simulink model "Model_3_Flux_weakening_control"  (R2017b)
settings: Solver=VariableStepAuto  StartTime=0.0  StopTime=5  MaxStep=1e-4  RelTol=1e-3  EnableMultiTasking=on
values from neighbouring files (symbols this model uses):
  Gain_I = 1    [Model_1_init.m]    (also in Model_2_init.m = 26.84; Model_3_init.m = 26.84)
  Gain_P = 1    [Model_1_init.m]    (also in Model_2_init.m = 7.74; Model_3_init.m = 7.74)
  Lambda_m = 0.2205    [Model_1_init.m]    (also in Model_2_init.m; Model_3_init.m)
  Ld = 1.7e-3    (= 0.0017)    [Model_1_init.m]    (also in Model_2_init.m; Model_3_init.m)
  Lq = 3.2e-3    (= 0.0032)    [Model_1_init.m]    (also in Model_2_init.m; Model_3_init.m)
  Param_BaseSpeed = 876    [Model_3_init.m]
  Param_Id_of_We_Torque = [0,-2.30177543036769,-8.59356944788153,-16.4990590457644,-24.2019970239658,-31.7336385477141,-39.1248735240059,-46.3895339353480,-53.5438693452557,-60.5877368527563,-67.5279121716960,-74.3632914076158,-81.0848264560473,-87.6900840096281,-94.1727155294297,-100.524695788491,-106.737943081073,-112.804868607954,-118.718887132852,-124.474863382221,-130.069470306117,-135.501440241541,-140.771697570859,- ...(+15575 chars)    [Model_3_init.m]
  Param_Iq_of_We_Torque = [0,17.4374754938312,33.6052724806698,47.9620946336906,61.0927552487034,73.1479215327095,84.3049660756008,94.6583419249824,104.337724889008,113.390978591554,121.917651973936,129.979877833255,137.614541014493,144.885610404097,151.839336396392,158.514190867132,164.945264651086,171.164425441937,177.200422756775,183.078971644055,188.822841517577,194.451970162672,199.983615838069,205.431863624177,210.80 ...(+14449 chars)    [Model_3_init.m]
  ParamControlTableTrqIndex = [0,23.5444010560252,47.0888021120504,70.6332031680755,94.1776042241007,117.722005280126,141.266406336151,164.810807392176,188.355208448201,211.899609504227,235.444010560252,258.988411616277,282.532812672302,306.077213728327,329.621614784353,353.166015840378,376.710416896403,400.254817952428,423.799219008453,447.343620064478,470.888021120504,494.432422176529,517.976823232554,541.521224288579,565.06 ...(+113 chars)    [Model_3_init.m]
  ParamControlTableWeIndex = [875.837524774747,1058.84332746136,1241.84913014798,1424.85493283460,1607.86073552121,1790.86653820783,1973.87234089444,2156.87814358106,2339.88394626768,2522.88974895429,2705.89555164091,2888.90135432753,3071.90715701414,3254.91295970076,3437.91876238737,3620.92456507399,3803.93036776061,3986.93617044722,4169.94197313384,4352.94777582045,4535.95357850707,4718.95938119369,4901.96518388030,5084.970 ...(+82 chars)    [Model_3_init.m]
  Polepairs = 4    [Model_1_init.m]    (also in Model_2_init.m; Model_3_init.m)
  Rs = 0.02    [Model_1_init.m]    (also in Model_2_init.m; Model_3_init.m)
undefined symbols (not defined in the file or in its folder): sigbuilder_block
libraries: powerlib x18, simulink x5, powerlib_meascontrol x1
settings Model: SimulationMode=accelerator  Creator=dakaihu  LastModifiedBy=proso
settings DataIOCC: LimitDataPoints=on
settings OptimizationCC: LifeSpan=inf
settings DebuggingCC: AllowSymbolicDim=off  SFUnexpectedBacktrackingDiag=warning  SFNoUnconditionalDefaultTransitionDiag=warning  SFExecutionAtInitializationDiag=none
settings ModelReferenceCC: PropagateSignalLabelsOutOfModel=off
settings CodeAppCC: StateflowObjectComments=on
settings GRTTargetCC: TargetLangStandard=C89/C90 (ANSI)
settings ConfigComp: CovMetricSettings=dw  CovSaveCumulativeToWorkspaceVar=on  CovSaveSingleToWorkspaceVar=on  CovExternalEMLEnable=off
settings SimscapeCC: SimscapeNormalizeSystem=off

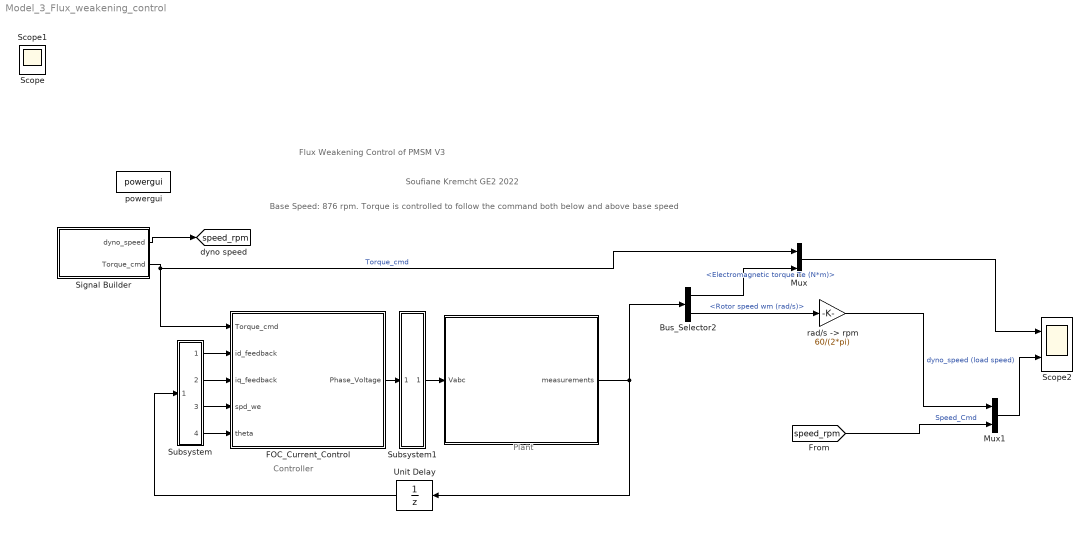
== system Model_3_Flux_weakening_control ==
  note: Soufiane Kremcht GE2 2022
  note: Base Speed: 876 rpm. Torque is controlled to follow the command both below and above base speed
  note: Controller
  note: Plant
  note: Flux Weakening Control of PMSM V3
  " " : Subsystem
  Bus_Selector2 : BusSelector  OutputSignals=Electromagnetic torque Te (N*m),Rotor speed wm (rad/s)
  FOC_Current_Control : Subsystem
  Mux : Mux  Inputs=2
  Mux1 : Mux  Inputs=2
  Scope2 : Scope  NumInputPorts=2
  Signal Builder : Subsystem  Tag=STV Subsys  LoadFcn=sigbuilder_block('load',[326.4 117 550.8 361.8 ]);  StartFcn=sigbuilder_block('start');  StopFcn=sigbuilder_block('stop');  ClipboardFcn=sigbuilder_block('clipboard');  mask(Sigbuilder block){tuvar=[0:10]}
      mask help: Simulink:masks:SigbuilderBlock_MD
      mask init:
      | if ~strcmp(get_param(bdroot(gcbh),'SimulationStatus'),'stopped') tuvar = sigbuilder_block('maskInit'); end
      settings: CopyFcn=sigbuilder_block('copy');  DeleteFcn=sigbuilder_block('delete');  ModelCloseFcn=sigbuilder_block('modelClose');  PreSaveFcn=sigbuilder_block('preSave');  PauseFcn=sigbuilder_block('pause');  ContinueFcn=sigbuilder_block('continue');  NameChangeFcn=sigbuilder_block('namechange');  OpenFcn=sigbuilder_block('open',[326.4 117 550.8 361.8 ]);  CloseFcn=sigbuilder_block('close');
      mask Display: plot(0, 0, 100, 100,[2, 2, 32, 32, 2], [68, 8, 8, 68, 68],[32, 2], [38, 38], [32, 19, 2],[53, 60, 44], [32, 17, 17, 2],[16, 16, 31, 31]);txt = getActiveGroup(gcbh);text(2, 100, txt,'verticalAlignment', 'top');
  Subsystem : Subsystem
      mask Display: fprintf('C/D')
  Subsystem1 : Subsystem
      mask Display: fprintf('D/C')
  Unit Delay : UnitDelay  SampleTime=1e-4
  powergui : powerlib/powergui  SimulationMode=Continuous  SampleTime=1e-5  frequency=60  Iterations=50  frequencyindice=0  Pbase=100e6  ErrMax=1e-4  UnitsV=kV  UnitsW=MW  buscounter=0  FunctionMessages=off  echomessages=off  EnableUseOfTLC=off  CurrentSourceSwitches=off  DisableSnubberDevices=off  DisableRonSwitches=off  DisableVfSwitches=off  DisplayEquations=off  SolverType=Tustin/Backward Euler (TBE)  Interpol=off  ExternalGateDelay=off  methode=off  Ts=100  x0status=blocks  SPID=on  SwTol=0  HookPort=off  RestoreLinks=warning  ResistiveCurrentMeasurement=off  Frange=[0:2:500]  Ylog=off  Xlog=on  ShowGrid=off  save=off  variable=ZData  structure=0  ZoomFFT=on  StartTime=0.0  cycles=1  DisplayStyle=1  fundamental=60  FreqAxis=off  MaxFrequency=1000  frequencyindicesteady=1  RmsSteady=1  display=off
  "rad/s -> rpm" : Gain  Gain=60/(2*pi)
  Scope : Scope
  Scope1 : Scope
  tag scope: speed_rpm=global
  wires:
  FOC_Current_Control/1(Phase_Voltage) -> Subsystem1/1(In1)
  " "/1(measurements) -> Unit Delay/1, Bus_Selector2/1
  Subsystem1/1(Out1) -> " "/1(Vabc)
  Unit Delay/1 -> Subsystem/1(PMSM_Measurements)
  Mux/1 -> Scope2/1
  Bus_Selector2/1 -> Mux/2  "<Electromagnetic torque Te (N*m)>"
  Subsystem/1(Out2) -> FOC_Current_Control/2(id_feedback)
  Subsystem/2(Out3) -> FOC_Current_Control/3(iq_feedback)
  Subsystem/3(Out1) -> FOC_Current_Control/4(spd_we)
  Subsystem/4(Out4) -> FOC_Current_Control/5(theta)
  Signal Builder/2(Torque_cmd) -> FOC_Current_Control/1(Torque_cmd), Mux/1  "Torque_cmd"
  Signal Builder/1(dyno_speed) -> [speed_rpm]
  Bus_Selector2/2 -> "rad/s -> rpm"/1  "<Rotor speed wm (rad/s)>"
  [speed_rpm] -> Mux1/2  "Speed_Cmd"
  "rad/s -> rpm"/1 -> Mux1/1  "dyno_speed (load speed)"
  Mux1/1 -> Scope2/2

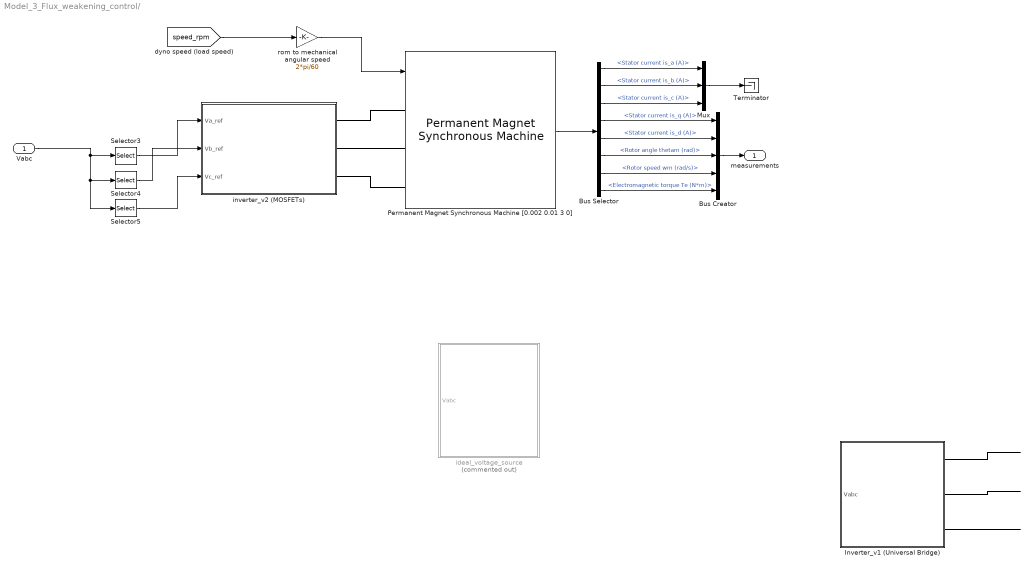
== system Model_3_Flux_weakening_control/  ==
  Vabc : Inport
  " Inverter_v1 (Universal Bridge)" : Subsystem
  Bus Creator : BusCreator  Inputs=5
  Bus Selector : BusSelector  OutputSignals=Stator current is_a (A),Stator current is_b (A),Stator current is_c (A),Stator current is_q (A),Stator current is_d (A),Rotor angle thetam (rad),Rotor speed wm (rad/s),Electromagnetic torque Te (N*m)
  Mux : Mux  Inputs=3
  Permanent Magnet Synchronous Machine [0.002 0.01 3 0] : powerlib/Machines/Permanent Magnet Synchronous Machine  NbPhases=3  FluxDistribution=Sinusoidal  RotorType=Salient-pole  MechanicalLoad=Speed w  PresetModel=No  ShowDetailedParameters=on  MeasurementBus=off  Resistance=Rs  Inductance=8.5e-3  dqInductances=[Ld,Lq]  La=0.000395  MachineConstant=Flux linkage established by magnets (V.s)  Flux=Lambda_m  VoltageCst=159.9771  TorqueCst=1.323  Flat=120  Mechanical=[0.0027 0.001 4 0]  PolePairs=Polepairs  InitialConditions=[0,0, 0,0]  InitialConditions5ph=[0 0 0 0 0 0]  TsPowergui=0  TsBlock=-1  RefAngle=Aligned with phase A axis (original Park)
  Selector3 : Selector  InputPortWidth=3  IndexOptions=Index vector (dialog)  Indices=[1]  OutputSizes=1
  Selector4 : Selector  InputPortWidth=3  IndexOptions=Index vector (dialog)  Indices=2  OutputSizes=1
  Selector5 : Selector  InputPortWidth=3  IndexOptions=Index vector (dialog)  Indices=3  OutputSizes=1
  Terminator : Terminator
  ideal_voltage_source : Subsystem  Commented=on  VariantControl=variantPwm == enumPwm.behavior
  inverter_v2 (MOSFETs) : Subsystem
  rom to mechanical angular speed : Gain  Gain=2*pi/60
  measurements : Outport
  wires:
  rom to mechanical angular speed/1 -> Permanent Magnet Synchronous Machine [0.002 0.01 3 0]/1
  Bus Selector/4 -> Bus Creator/1  "<Stator current is_q (A)>"
  Bus Selector/5 -> Bus Creator/2  "<Stator current is_d (A)>"
  Bus Selector/6 -> Bus Creator/3  "<Rotor angle thetam (rad)>"
  Bus Creator/1 -> measurements/1
  Bus Selector/1 -> Mux/1  "<Stator current is_a (A)>"
  Bus Selector/2 -> Mux/2  "<Stator current is_b (A)>"
  Bus Selector/3 -> Mux/3  "<Stator current is_c (A)>"
  Mux/1 -> Terminator/1
  Permanent Magnet Synchronous Machine [0.002 0.01 3 0]/1 -> Bus Selector/1
  Bus Selector/7 -> Bus Creator/4  "<Rotor speed wm (rad/s)>"
  [speed_rpm] -> rom to mechanical angular speed/1
  Bus Selector/8 -> Bus Creator/5  "<Electromagnetic torque Te (N*m)>"
  Vabc/1 -> Selector5/1, Selector4/1, Selector3/1
  Selector3/1 -> inverter_v2 (MOSFETs)/1(Va_ref)
  Selector4/1 -> inverter_v2 (MOSFETs)/2(Vb_ref)
  Selector5/1 -> inverter_v2 (MOSFETs)/3(Vc_ref)
  connections:
  " Inverter_v1 (Universal Bridge)"/RConn3 -- ?
  " Inverter_v1 (Universal Bridge)"/RConn2 -- ?
  " Inverter_v1 (Universal Bridge)"/RConn1 -- ?
  inverter_v2 (MOSFETs)/RConn1 -- Permanent Magnet Synchronous Machine [0.002 0.01 3 0]/LConn1
  inverter_v2 (MOSFETs)/RConn2 -- Permanent Magnet Synchronous Machine [0.002 0.01 3 0]/LConn2
  inverter_v2 (MOSFETs)/RConn3 -- Permanent Magnet Synchronous Machine [0.002 0.01 3 0]/LConn3

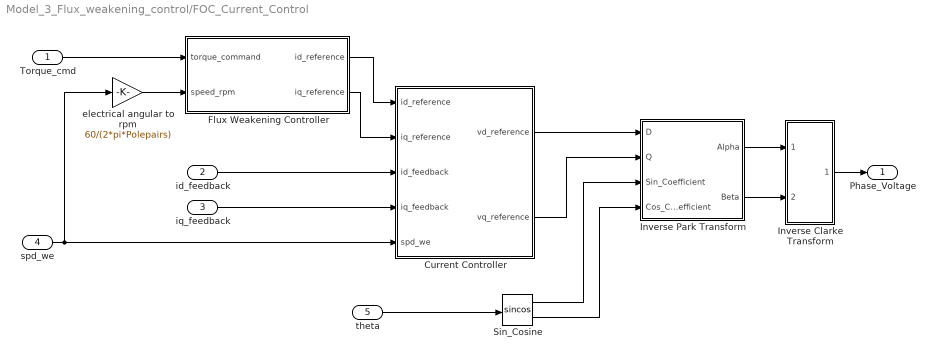
== system Model_3_Flux_weakening_control/FOC_Current_Control ==
  Torque_cmd : Inport
  id_feedback : Inport  Port=2
  iq_feedback : Inport  Port=3
  spd_we : Inport  Port=4
  theta : Inport  Port=5
  Current Controller : Subsystem
  Flux Weakening Controller : Subsystem
  Inverse Clarke Transform : Subsystem
  Inverse Park Transform : Subsystem
  Sin_Cosine : Trigonometry  Operator=sincos
  electrical angular to rpm : Gain  Gain=60/(2*pi*Polepairs)
  Phase_Voltage : Outport  SampleTime=1e-4
  wires:
  Inverse Clarke Transform/1(ABC) -> Phase_Voltage/1
  Sin_Cosine/2 -> Inverse Park Transform/4(Cos_Coefficient)
  Sin_Cosine/1 -> Inverse Park Transform/3(Sin_Coefficient)
  theta/1 -> Sin_Cosine/1
  Current Controller/2(vq_reference) -> Inverse Park Transform/2(Q)
  Current Controller/1(vd_reference) -> Inverse Park Transform/1(D)
  Inverse Park Transform/1(Alpha) -> Inverse Clarke Transform/1(Alpha)
  Inverse Park Transform/2(Beta) -> Inverse Clarke Transform/2(Beta)
  Flux Weakening Controller/1(id_reference) -> Current Controller/1(id_reference)
  Flux Weakening Controller/2(iq_reference) -> Current Controller/2(iq_reference)
  Torque_cmd/1 -> Flux Weakening Controller/1(torque_command)
  spd_we/1 -> Current Controller/5(spd_we), electrical angular to rpm/1
  electrical angular to rpm/1 -> Flux Weakening Controller/2(speed_rpm)
  id_feedback/1 -> Current Controller/3(id_feedback)
  iq_feedback/1 -> Current Controller/4(iq_feedback)

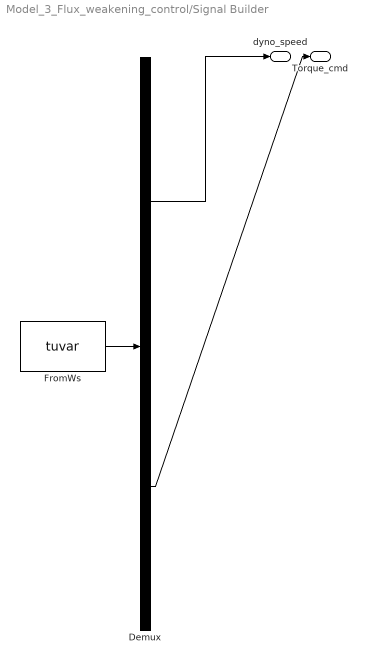
== system Model_3_Flux_weakening_control/Signal Builder ==
  Demux : Demux  Tag=STV Demux  Outputs=2
  FromWs : FromWorkspace  Tag=STV FromWs  VariableName=tuvar  SampleTime=0
      SigBuilderData=|
      | common.afterFinalStr = 'Extrapolate'
      | common.sampleTime = 0
      | dataSet.timeRange = [0 3]
      | dataSet.name = 'Group 1'
      | sbobj.Groups.Name = 'Group 1'
      | sbobj.Groups.Signals(1).Name = 'dyno_speed'
      | sbobj.Groups.Signals(1).XData = [0 1 2 3]
      | sbobj.Groups.Signals(1).YData = [0 1500 1500 -20]
      | sbobj.Groups.Signals(2).Name = 'Torque_cmd'
      | sbobj.Groups.Signals(2).XData = [0 0.995 0.995 3]
      | sbobj.Groups.Signals(2).YData = [100 98 218 218]
      | sbobj.Groups.TimeRange = [0 3]
  dyno_speed : Outport  Tag=STV Outport
  Torque_cmd : Outport  Tag=STV Outport  Port=2
  wires:
  Demux/1 -> dyno_speed/1
  FromWs/1 -> Demux/1
  Demux/2 -> Torque_cmd/1

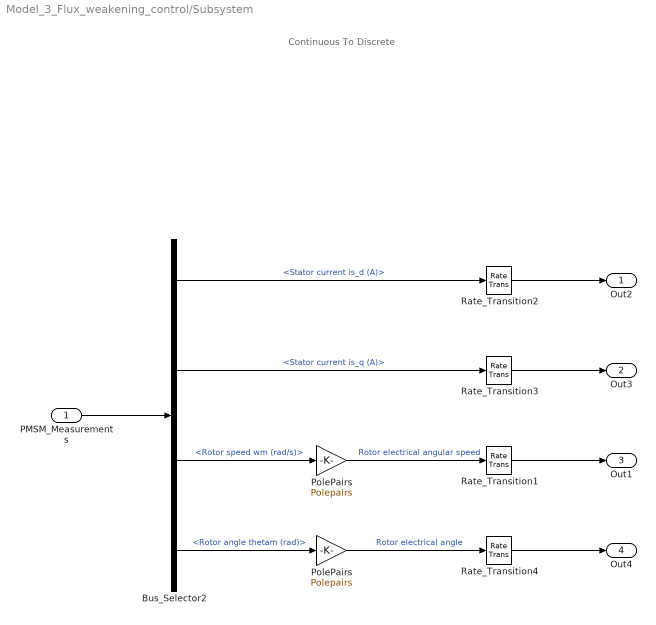
== system Model_3_Flux_weakening_control/Subsystem ==
  note: Continuous To Discrete
  PMSM_Measurements : Inport
  Bus_Selector2 : BusSelector  OutputSignals=Stator current is_d (A),Stator current is_q (A),Rotor speed wm (rad/s),Rotor angle thetam (rad)
  PolePairs : Gain  Gain=Polepairs
  "PolePairs " : Gain  Gain=Polepairs
  Rate_Transition{1..4} (4 alike) : RateTransition  Integrity=off  Deterministic=off
  Out2 : Outport
  Out3 : Outport  Port=2
  Out1 : Outport  Port=3
  Out4 : Outport  Port=4
  wires:
  Rate_Transition4/1 -> Out4/1
  Bus_Selector2/4 -> PolePairs/1  "<Rotor angle thetam (rad)>"
  PMSM_Measurements/1 -> Bus_Selector2/1
  PolePairs/1 -> Rate_Transition4/1  "Rotor electrical angle"
  Rate_Transition2/1 -> Out2/1
  Rate_Transition3/1 -> Out3/1
  Rate_Transition1/1 -> Out1/1
  Bus_Selector2/3 -> "PolePairs "/1  "<Rotor speed wm (rad/s)>"
  "PolePairs "/1 -> Rate_Transition1/1  "Rotor electrical angular speed"
  Bus_Selector2/1 -> Rate_Transition2/1  "<Stator current is_d (A)>"
  Bus_Selector2/2 -> Rate_Transition3/1  "<Stator current is_q (A)>"

== system Model_3_Flux_weakening_control/Subsystem1 ==
  In1 : Inport
  Rate_Transition1 : RateTransition  Integrity=off
  Out1 : Outport
  wires:
  In1/1 -> Rate_Transition1/1
  Rate_Transition1/1 -> Out1/1

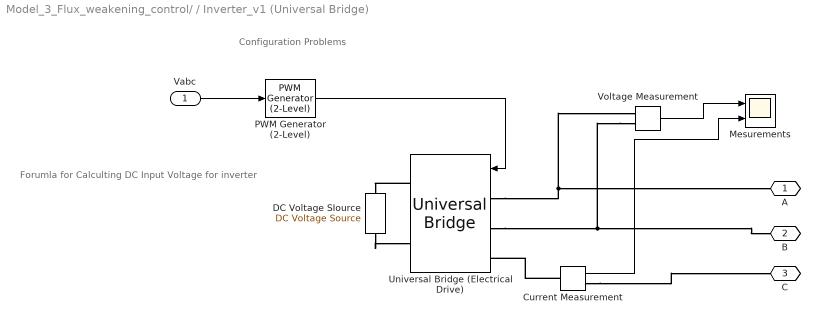
== system Model_3_Flux_weakening_control/ / Inverter_v1 (Universal Bridge) ==
  note: Forumla for Calculting DC Input Voltage for inverter
  note: Configuration Problems
  Vabc : Inport
  Current Measurement : powerlib/Measurements/Current Measurement  PhasorSimulation=off  OutputType=Complex  PSBequivalent=0
  DC Voltage SIource : powerlib/Electrical Sources/DC Voltage Source  Amplitude=320  Measurements=None
  Mesurements : Scope  NumInputPorts=2
  PWM Generator (2-Level) : powerlib_meascontrol/Pulse & Signal Generators/PWM Generator (2-Level)  ModulatorType=Three-phase bridge (6 pulses)  ModulatorMode=Unsynchronized  Fc=27*60  Pc=90  nF=27  MinMax="[ -1  1 ]"  SamplingTechnique=Natural  ModulatingSignals=off  m=0.8  Freq=60  Phase=0  Ts=0  ShowCarrierOutport=off
      settings: SourceProductName=Simscape Power Systems
  Universal Bridge (Electrical Drive) : powerlib/Power Electronics/Universal Bridge  Arms=3  SnubberResistance=1e5  SnubberCapacitance=inf  Device=IGBT / Diodes  Ron=1e-2  Lon=0  ForwardVoltages="[  0  0  ]"  ForwardVoltage=0  GTOparameters=[ 10e-6 , 20e-6 ]  IGBTparameters=[ 1e-6 , 2e-6 ]  Measurements=None  Measurements_2=None  converterType=Rectifier
  Voltage Measurement : powerlib/Measurements/Voltage Measurement  PhasorSimulation=off  OutputType=Complex  PSBequivalent=0
  A : PMIOPort  Port=1  Side=Right
  B : PMIOPort  Port=2  Side=Right
  C : PMIOPort  Port=3  Side=Right
  wires:
  PWM Generator (2-Level)/1 -> Universal Bridge (Electrical Drive)/1
  Vabc/1 -> PWM Generator (2-Level)/1
  Voltage Measurement/1 -> Mesurements/1
  Current Measurement/1 -> Mesurements/2
  connections:
  Universal Bridge (Electrical Drive)/RConn1 -- DC Voltage SIource/RConn1
  DC Voltage SIource/LConn1 -- Universal Bridge (Electrical Drive)/RConn2
  Current Measurement/LConn1 -- Universal Bridge (Electrical Drive)/LConn3
  Universal Bridge (Electrical Drive)/LConn1 -- Voltage Measurement/LConn1 -- A/RConn1
  Voltage Measurement/LConn2 -- Universal Bridge (Electrical Drive)/LConn2 -- B/RConn1
  Current Measurement/RConn1 -- C/RConn1

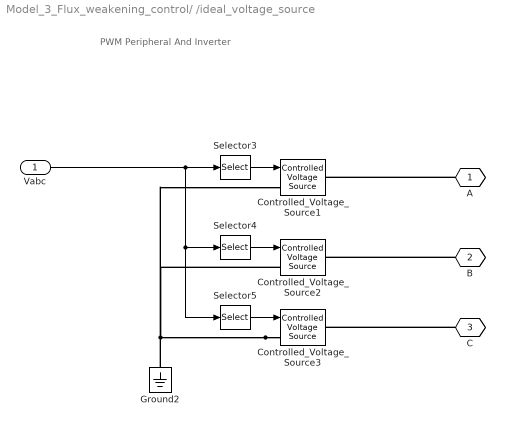
== system Model_3_Flux_weakening_control/ /ideal_voltage_source ==
  note: PWM Peripheral And Inverter
  Vabc : Inport
  Controlled_Voltage_Source1 : powerlib/Electrical Sources/Controlled Voltage Source  Initialize=off  Source_Type=DC  Amplitude=12  Phase=0  Frequency=0  Measurements=None
  Controlled_Voltage_Source2 : powerlib/Electrical Sources/Controlled Voltage Source  Initialize=off  Source_Type=DC  Amplitude=12  Phase=0  Frequency=0  Measurements=None
  Controlled_Voltage_Source3 : powerlib/Electrical Sources/Controlled Voltage Source  Initialize=off  Source_Type=DC  Amplitude=12  Phase=0  Frequency=0  Measurements=None
  Ground2 : powerlib/Elements/Ground  LConnTagsString=a
  Selector3 : Selector  InputPortWidth=3  IndexOptions=Index vector (dialog)  Indices=[1]  OutputSizes=1
  Selector4 : Selector  InputPortWidth=3  IndexOptions=Index vector (dialog)  Indices=2  OutputSizes=1
  Selector5 : Selector  InputPortWidth=3  IndexOptions=Index vector (dialog)  Indices=3  OutputSizes=1
  A : PMIOPort  Tag=PMCPort  Port=1  Side=Right
  B : PMIOPort  Tag=PMCPort  Port=2  Side=Right
  C : PMIOPort  Tag=PMCPort  Port=3  Side=Right
  wires:
  Vabc/1 -> Selector4/1, Selector5/1, Selector3/1
  Selector5/1 -> Controlled_Voltage_Source3/1
  Selector4/1 -> Controlled_Voltage_Source2/1
  Selector3/1 -> Controlled_Voltage_Source1/1
  connections:
  C/RConn1 -- Controlled_Voltage_Source3/RConn1
  B/RConn1 -- Controlled_Voltage_Source2/RConn1
  A/RConn1 -- Controlled_Voltage_Source1/RConn1
  Controlled_Voltage_Source3/LConn1 -- Controlled_Voltage_Source1/LConn1 -- Controlled_Voltage_Source2/LConn1 -- Ground2/LConn1

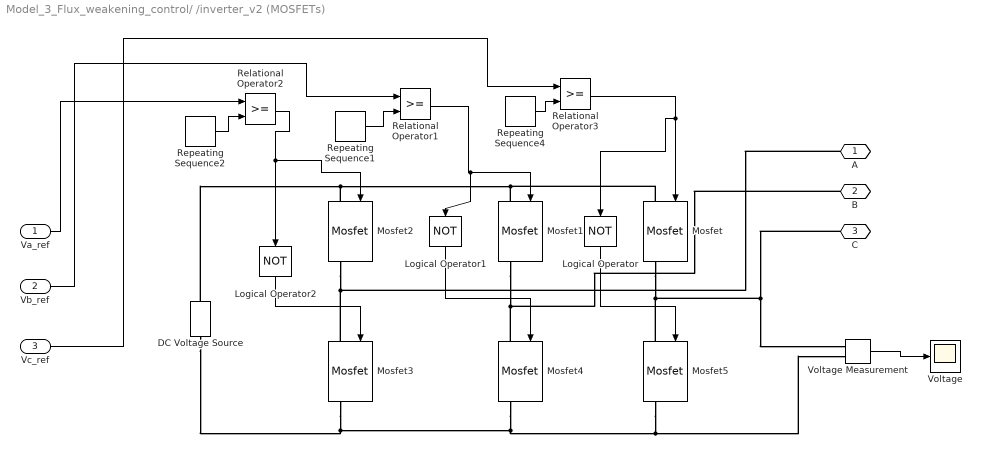
== system Model_3_Flux_weakening_control/ /inverter_v2 (MOSFETs) ==
  Va_ref : Inport
  Vb_ref : Inport  Port=2
  Vc_ref : Inport  Port=3
  DC Voltage Source : powerlib/Electrical Sources/DC Voltage Source  Amplitude=320  Measurements=None
  Logical Operator : Logic  Operator=NOT  AllPortsSameDT=off  OutDataTypeStr=boolean
  Logical Operator1 : Logic  Operator=NOT  AllPortsSameDT=off  OutDataTypeStr=boolean
  Logical Operator2 : Logic  Operator=NOT  AllPortsSameDT=off  OutDataTypeStr=boolean
  Mosfet{,1..5} (6 alike) : powerlib/Power Electronics/Mosfet  Ron=0.1  Lon=0  Rd=0.01  Vfd=0  IC=0  Rs=1e5  Cs=inf  Measurements=on
  Relational Operator1 : RelationalOperator  OutDataTypeStr=boolean  RndMeth=Simplest
  Relational Operator2 : RelationalOperator  OutDataTypeStr=boolean  RndMeth=Simplest
  Relational Operator3 : RelationalOperator  OutDataTypeStr=boolean  RndMeth=Simplest
  Repeating Sequence1 : simulink/Sources/Repeating Sequence  rep_seq_t="[0 (1/5000)/4  (1/5000)/2 (3/5000)/4 1/5000]"  rep_seq_y=[0 1 0 -1 0]
  Repeating Sequence2 : simulink/Sources/Repeating Sequence  rep_seq_t="[0 (1/5000)/4  (1/5000)/2 (3/5000)/4 1/5000]"  rep_seq_y=[0 1 0 -1 0]
  Repeating Sequence4 : simulink/Sources/Repeating Sequence  rep_seq_t="[0 (1/5000)/4  (1/5000)/2 (3/5000)/4 1/5000]"  rep_seq_y=[0 1 0 -1 0]
  Voltage : Scope
  Voltage Measurement : powerlib/Measurements/Voltage Measurement  PhasorSimulation=off  OutputType=Complex  PSBequivalent=0
  A : PMIOPort  Port=1  Side=Right
  B : PMIOPort  Port=2  Side=Right
  C : PMIOPort  Port=3  Side=Right
  wires:
  Relational Operator1/1 -> Mosfet1/1, Logical Operator1/1
  Vc_ref/1 -> Relational Operator3/1
  Logical Operator2/1 -> Mosfet3/1
  Va_ref/1 -> Relational Operator2/1
  Repeating Sequence4/1 -> Relational Operator3/2
  Repeating Sequence2/1 -> Relational Operator2/2
  Repeating Sequence1/1 -> Relational Operator1/2
  Relational Operator3/1 -> Mosfet/1, Logical Operator/1
  Relational Operator2/1 -> Mosfet2/1, Logical Operator2/1
  Vb_ref/1 -> Relational Operator1/1
  Logical Operator/1 -> Mosfet5/1
  Logical Operator1/1 -> Mosfet4/1
  Voltage Measurement/1 -> Voltage/1
  connections:
  Mosfet2/LConn1 -- Mosfet1/LConn1 -- Mosfet/LConn1 -- DC Voltage Source/RConn1
  Mosfet5/LConn1 -- Mosfet/RConn1 -- C/RConn1 -- Voltage Measurement/LConn1
  Mosfet3/LConn1 -- Mosfet2/RConn1 -- A/RConn1
  Mosfet5/RConn1 -- DC Voltage Source/LConn1 -- Mosfet3/RConn1 -- Mosfet4/RConn1 -- Voltage Measurement/LConn2
  Mosfet4/LConn1 -- Mosfet1/RConn1 -- B/RConn1

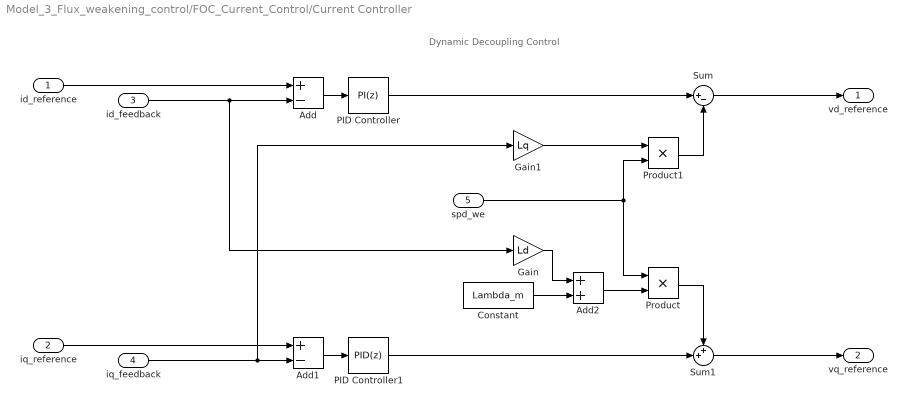
== system Model_3_Flux_weakening_control/FOC_Current_Control/Current Controller ==
  note: Dynamic Decoupling Control
  id_reference : Inport  SampleTime=1e-4
  iq_reference : Inport  Port=2  SampleTime=1e-4
  id_feedback : Inport  Port=3  SampleTime=1e-4
  iq_feedback : Inport  Port=4  SampleTime=1e-4
  spd_we : Inport  Port=5  SampleTime=1e-4
  Add : Sum  Inputs=+-
  Add1 : Sum  Inputs=+-
  Add2 : Sum
  Constant : Constant  Value=Lambda_m  SampleTime=1e-4
  Gain : Gain  Gain=Ld
  Gain1 : Gain  Gain=Lq
  PID Controller : simulink/Continuous/PID Controller  Controller=PI  TimeDomain=Discrete-time  SampleTime=-1  IntegratorMethod=Forward Euler  FilterMethod=Forward Euler  Form=Parallel  UseFilter=on  ControllerParametersSource=internal  P=Gain_P  I=Gain_I  D=0  N=100  InitialConditionSource=internal  InitialConditionForIntegrator=0  InitialConditionForFilter=0  ExternalReset=none  LimitOutput=off  UpperSaturationLimit=inf  LowerSaturationLimit=-inf  LinearizeAsGain=on  AntiWindupMode=none  Kb=1  TrackingMode=off  Kt=1  PParamMin=[]  PParamMax=[]  IParamMin=[]  IParamMax=[]  DParamMin=[]  DParamMax=[]  NParamMin=[]  NParamMax=[]  KbParamMin=[]  KbParamMax=[]  KtParamMin=[]  KtParamMax=[]  POutMin=[]  POutMax=[]  IOutMin=[]  IOutMax=[]  DOutMin=[]  DOutMax=[]  NOutMin=[]  NOutMax=[]  KbOutMin=[]  KbOutMax=[]  KtOutMin=[]  KtOutMax=[]  IntegratorOutMin=[]  IntegratorOutMax=[]  FilterOutMin=[]  FilterOutMax=[]  SumOutMin=[]  SumOutMax=[]  SumI1OutMin=[]  SumI1OutMax=[]  SumI2OutMin=[]  SumI2OutMax=[]  SumI3OutMin=[]  SumI3OutMax=[]  SumDOutMin=[]  SumDOutMax=[]  SaturationOutMin=[]  SaturationOutMax=[]  IntegratorContinuousStateAttributes=''  IntegratorStateMustResolveToSignalObject=off  IntegratorRTWStateStorageClass=Auto  FilterContinuousStateAttributes=''  FilterStateMustResolveToSignalObject=off  FilterRTWStateStorageClass=Auto  DifferentiatorICPrevScaledInput=0  DifferentiatorOutMin=[]  DifferentiatorOutMax=[]  InitialConditionSetting=State (most efficient)  FilterDiffOutCoefMin=[]  FilterDiffOutCoefMax=[]  SumDenOutMin=[]  SumDenOutMax=[]  SumNumOutMin=[]  SumNumOutMax=[]  ReciprocalOutMin=[]  ReciprocalOutMax=[]  DivideOutMin=[]  DivideOutMax=[]  TunerSelectOption=Transfer Function Based (PID Tuner App)
  PID Controller1 : simulink/Continuous/PID Controller  Controller=PID  TimeDomain=Discrete-time  SampleTime=-1  IntegratorMethod=Forward Euler  FilterMethod=Forward Euler  Form=Parallel  UseFilter=on  ControllerParametersSource=internal  P=Gain_P  I=Gain_I  D=0  N=100  InitialConditionSource=internal  InitialConditionForIntegrator=0  InitialConditionForFilter=0  ExternalReset=none  LimitOutput=off  UpperSaturationLimit=inf  LowerSaturationLimit=-inf  LinearizeAsGain=on  AntiWindupMode=none  Kb=1  TrackingMode=off  Kt=1  PParamMin=[]  PParamMax=[]  IParamMin=[]  IParamMax=[]  DParamMin=[]  DParamMax=[]  NParamMin=[]  NParamMax=[]  KbParamMin=[]  KbParamMax=[]  KtParamMin=[]  KtParamMax=[]  POutMin=[]  POutMax=[]  IOutMin=[]  IOutMax=[]  DOutMin=[]  DOutMax=[]  NOutMin=[]  NOutMax=[]  KbOutMin=[]  KbOutMax=[]  KtOutMin=[]  KtOutMax=[]  IntegratorOutMin=[]  IntegratorOutMax=[]  FilterOutMin=[]  FilterOutMax=[]  SumOutMin=[]  SumOutMax=[]  SumI1OutMin=[]  SumI1OutMax=[]  SumI2OutMin=[]  SumI2OutMax=[]  SumI3OutMin=[]  SumI3OutMax=[]  SumDOutMin=[]  SumDOutMax=[]  SaturationOutMin=[]  SaturationOutMax=[]  IntegratorContinuousStateAttributes=''  IntegratorStateMustResolveToSignalObject=off  IntegratorRTWStateStorageClass=Auto  FilterContinuousStateAttributes=''  FilterStateMustResolveToSignalObject=off  FilterRTWStateStorageClass=Auto  DifferentiatorICPrevScaledInput=0  DifferentiatorOutMin=[]  DifferentiatorOutMax=[]  InitialConditionSetting=State (most efficient)  FilterDiffOutCoefMin=[]  FilterDiffOutCoefMax=[]  SumDenOutMin=[]  SumDenOutMax=[]  SumNumOutMin=[]  SumNumOutMax=[]  ReciprocalOutMin=[]  ReciprocalOutMax=[]  DivideOutMin=[]  DivideOutMax=[]  TunerSelectOption=Transfer Function Based (PID Tuner App)
  Product : Product
  Product1 : Product
  Sum : Sum  Inputs=|+-
  Sum1 : Sum  Inputs=++|
  vd_reference : Outport  SampleTime=1e-4
  vq_reference : Outport  Port=2  SampleTime=1e-4
  wires:
  Sum/1 -> vd_reference/1
  PID Controller/1 -> Sum/1
  id_feedback/1 -> Gain/1, Add/2
  Add/1 -> PID Controller/1
  iq_feedback/1 -> Gain1/1, Add1/2
  id_reference/1 -> Add/1
  Add1/1 -> PID Controller1/1
  iq_reference/1 -> Add1/1
  Sum1/1 -> vq_reference/1
  PID Controller1/1 -> Sum1/2
  Gain/1 -> Add2/1
  Constant/1 -> Add2/2
  Add2/1 -> Product/2
  spd_we/1 -> Product1/2, Product/1
  Gain1/1 -> Product1/1
  Product1/1 -> Sum/2
  Product/1 -> Sum1/1

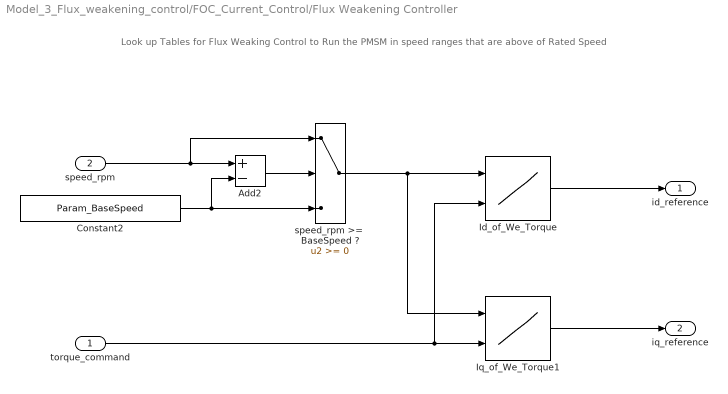
== system Model_3_Flux_weakening_control/FOC_Current_Control/Flux Weakening Controller ==
  note: Look up Tables for Flux Weaking Control to Run the PMSM in speed ranges that are above of Rated Speed
  torque_command : Inport  SampleTime=1e-4
  speed_rpm : Inport  Port=2  SampleTime=1e-4
  Add2 : Sum  Inputs=+-
  Constant2 : Constant  Value=Param_BaseSpeed  SampleTime=1e-4
  Id_of_We_Torque : Lookup_n-D  BreakpointsForDimension1=ParamControlTableWeIndex  BreakpointsForDimension2=ParamControlTableTrqIndex  Table=Param_Id_of_We_Torque  InternalRulePriority=Speed  RndMeth=Simplest  InputSameDT=on
  Iq_of_We_Torque1 : Lookup_n-D  BreakpointsForDimension1=ParamControlTableWeIndex  BreakpointsForDimension2=ParamControlTableTrqIndex  Table=Param_Iq_of_We_Torque  InternalRulePriority=Speed  RndMeth=Simplest  InputSameDT=on
  speed_rpm >=  BaseSpeed ? : Switch
  id_reference : Outport  SampleTime=1e-4
  iq_reference : Outport  Port=2  SampleTime=1e-4
  wires:
  Constant2/1 -> speed_rpm >=  BaseSpeed ?/3, Add2/2
  speed_rpm >=  BaseSpeed ?/1 -> Iq_of_We_Torque1/1, Id_of_We_Torque/1
  Id_of_We_Torque/1 -> id_reference/1
  Add2/1 -> speed_rpm >=  BaseSpeed ?/2
  speed_rpm/1 -> speed_rpm >=  BaseSpeed ?/1, Add2/1
  Iq_of_We_Torque1/1 -> iq_reference/1
  torque_command/1 -> Iq_of_We_Torque1/2, Id_of_We_Torque/2

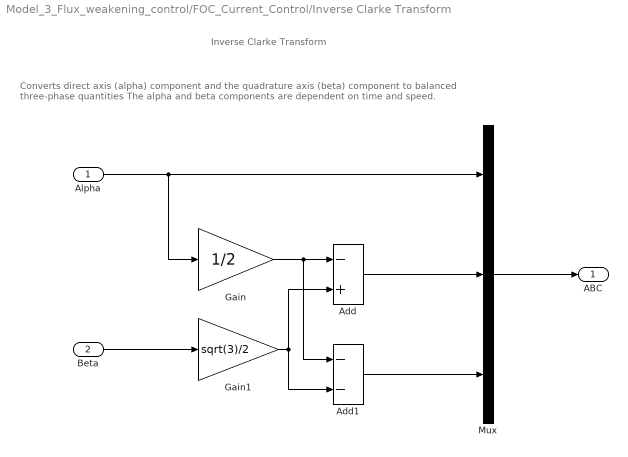
== system Model_3_Flux_weakening_control/FOC_Current_Control/Inverse Clarke Transform ==
  note: Inverse Clarke Transform
  note: Converts direct axis (alpha) component and the quadrature axis (beta) component to balanced three-phase quantities
      | The alpha and beta components are dependent on time and speed.
  Alpha : Inport
  Beta : Inport  Port=2
  Add : Sum  Inputs=-+  OutDataTypeStr=Inherit: Same as first input
  Add1 : Sum  Inputs=--  OutDataTypeStr=Inherit: Same as first input
  Gain : Gain  Gain=1/2
  Gain1 : Gain  Gain=sqrt(3)/2
  Mux : Mux  Inputs=3
  ABC : Outport
  wires:
  Beta/1 -> Gain1/1
  Mux/1 -> ABC/1
  Alpha/1 -> Mux/1, Gain/1
  Add1/1 -> Mux/3
  Gain1/1 -> Add1/2, Add/2
  Gain/1 -> Add1/1, Add/1
  Add/1 -> Mux/2

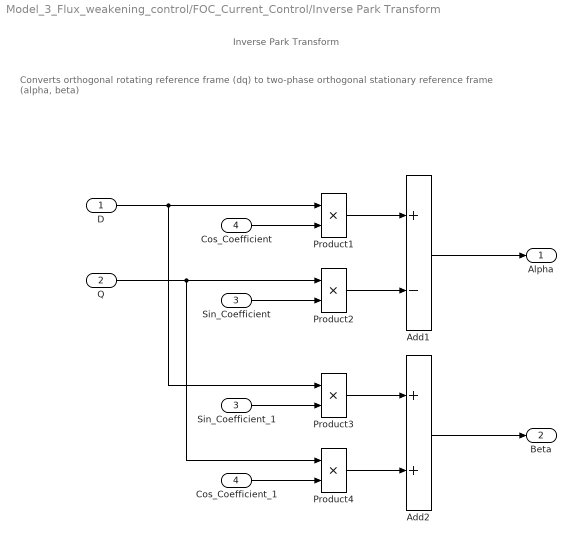
== system Model_3_Flux_weakening_control/FOC_Current_Control/Inverse Park Transform ==
  note: Converts orthogonal rotating reference frame (dq) to two-phase orthogonal stationary reference frame (alpha, beta)
  note: Inverse Park Transform
  D : Inport
  Q : Inport  Port=2
  Sin_Coefficient : Inport  Port=3
  Cos_Coefficient : Inport  Port=4
  Add1 : Sum  Inputs=+-  OutDataTypeStr=Inherit: Same as first input
  Add2 : Sum  OutDataTypeStr=Inherit: Same as first input
  Cos_Coefficient_1 : InportShadow  Port=4
  Product{1..4} (4 alike) : Product  RndMeth=Simplest
  Sin_Coefficient_1 : InportShadow  Port=3
  Alpha : Outport
  Beta : Outport  Port=2
  wires:
  Sin_Coefficient_1/1 -> Product3/2
  Product2/1 -> Add1/2
  Cos_Coefficient_1/1 -> Product4/2
  Add2/1 -> Beta/1
  Product3/1 -> Add2/1
  Add1/1 -> Alpha/1
  Product1/1 -> Add1/1
  Product4/1 -> Add2/2
  Sin_Coefficient/1 -> Product2/2
  D/1 -> Product3/1, Product1/1
  Q/1 -> Product2/1, Product4/1
  Cos_Coefficient/1 -> Product1/2
